simulink model "simulink_inline"  (Simulink 7.9)
settings: Solver=FixedStepDiscrete  StartTime=0.0  StopTime=10.0  RelTol=1e-3  SampleTimeConstraint=STIndependent
PreLoadFcn:
  | rtwdemo_paraminline_data
undefined symbols (not defined in the file or in its folder): MAX_LIFT, SLIDER_POS, T1Break, T1Data, T2Break, T2Data
libraries: rtwdemowidgets x3
Description:
  | Inlining Block Parameters and Propagating Constant Values
settings Model: Creator=The MathWorks Inc.  LastModifiedBy=boakes  CovMetricSettings=d  ExtModeAutoUpdateStatusClock=off
settings DataIOCC: SaveOutput=off  SaveTime=off  SignalLoggingName=sigsOut
settings OptimizationCC: InlineParams=on  InlineInvariantSignals=on  StateBitsets=on  DataBitsets=on  UseTempVars=on  EfficientFloat2IntCast=on  EfficientMapNaN2IntZero=off
settings DebuggingCC: CheckExecutionContextPreStartOutputMsg=on  CheckExecutionContextRuntimeOutputMsg=on  SolverPrmCheckMsg=none  FcnCallInpInsideContextMsg=Use local settings  StrictBusMsg=ErrorOnBusTreatedAsVector
settings HardwareCC: ProdIntDivRoundTo=Zero  ProdEndianess=LittleEndian  ProdHWDeviceType=Generic->32-bit Embedded Processor  TargetHWDeviceType=Generic->32-bit Embedded Processor
settings RTWCC: TLCOptions=-p0 -aWarnNonSaturatedBlocks=0  GenerateReport=on  RTWVerbose=off  ProcessScript=grt_make_rtw_hook  LaunchReport=on
settings CodeAppCC: ForceParamTrailComments=on
settings GRTTargetCC: TargetFcnLib=ansi_tfl_tmw.mat  UtilityFuncGeneration=Shared location

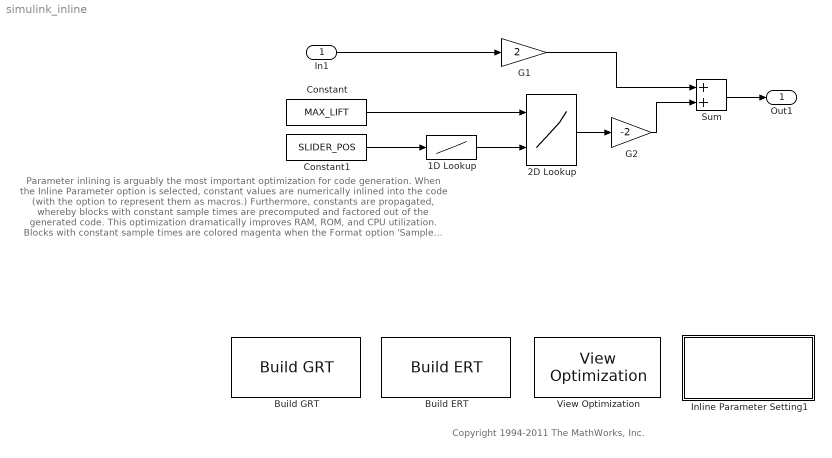
== system simulink_inline ==
  note: Parameter inlining is arguably the most important optimization for code generation.
      | When the Inline Parameter option is selected, constant values are numerically inlined
      | into the code (with the option to represent them as macros.)  Furthermore, constants are
      | propagated, whereby blocks with constant sample times are precomputed and factored
      | out of the generated code.  This optimization dramatically improves RAM, ROM, and
      | CPU utilization.  Blocks with constant sample times are colored magenta when the Format
      | option 'Sample Time Colors' is selected.
  note: Copyright 1994-2011 The MathWorks, Inc.
  In1 : Inport  OutDataTypeStr=double  PortDimensions=1
  1D Lookup : Lookup_n-D  NumberOfTableDimensions=1  BreakpointsForDimension1=T1Break  Table=T1Data  SaturateOnIntegerOverflow=on  InputSameDT=on
  2D Lookup : Lookup_n-D  BreakpointsForDimension1=T2Break  BreakpointsForDimension2=T2Break  Table=T2Data  InputSameDT=on
  Build ERT : rtwdemowidgets/Build ERT  attrib_overrides={}
  Build GRT : rtwdemowidgets/Build GRT  attrib_overrides={}
  Constant : Constant  Value=MAX_LIFT
  Constant1 : Constant  Value=SLIDER_POS
  G1 : Gain  Gain=2  SaturateOnIntegerOverflow=on  OutDataTypeStr=Inherit: Same as input  ParamDataTypeStr=Inherit: Same as input
  G2 : Gain  Gain=-2  SaturateOnIntegerOverflow=on  OutDataTypeStr=Inherit: Same as input  ParamDataTypeStr=Inherit: Same as input
  Inline Parameter Setting1 : Subsystem
      settings: OpenFcn=m=get_param(bdroot,'name'); set_param(bdroot, 'SampleTimeColors','on'); eval([m,'([],[],[],''compile'');']); eval([m,'([],[],[],''term'');']); clear m;
      mask Display: disp(sprintf('Display Sample\nTime Colors\n(double-click)'))
  Sum : Sum
  View Optimization : rtwdemowidgets/View Optimization  SystemSampleTime=-1
  Out1 : Outport
  wires:
  In1/1 -> G1/1
  Sum/1 -> Out1/1
  Constant/1 -> 2D Lookup/1
  Constant1/1 -> 1D Lookup/1
  1D Lookup/1 -> 2D Lookup/2
  2D Lookup/1 -> G2/1
  G1/1 -> Sum/1
  G2/1 -> Sum/2

== system simulink_inline/Inline Parameter Setting1 ==
